simulink model "step2-part3"  (R2020b)
settings: Solver=VariableStepAuto  StartTime=0.0  StopTime=20  RelTol=1e-3
libraries: dspsnks4 x1, dspsrcs4 x1, dspvision x1, dspadpt3 x1
settings Model: Creator=berkt  LastModifiedBy=berkt

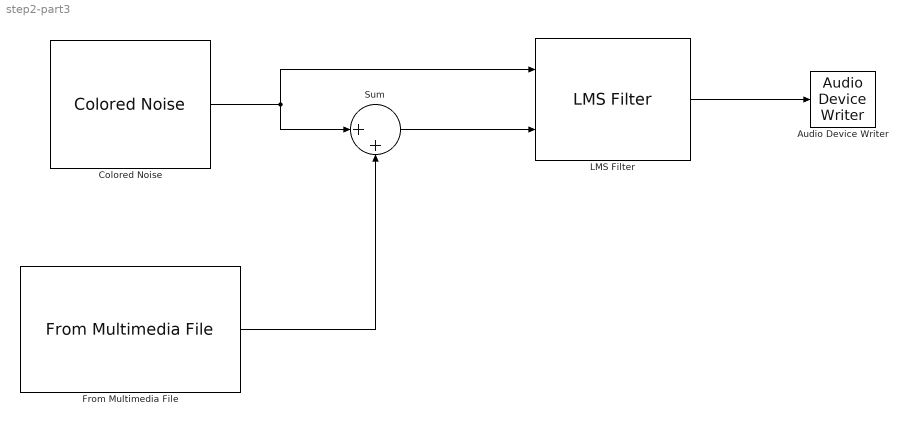
== system step2-part3 ==
  Audio Device Writer : dspsnks4/Audio Device Writer  Driver=DirectSound  Device=Default  InheritSampleRate=on  SampleRate=44100  BitDepth=16-bit integer  BufferSize=4096  NumBuffers=10  DefaultOutputChannelMapping=on  OutputChannelMapping=1:2  OutputNumUnderrunSamples=off  DriverIdx=1  DeviceWarnFlag=''
  Colored Noise : dspsrcs4/Colored Noise  Color=pink  InverseFrequencyPower=1  BoundedOutput=on  NumChannels=1  OutputDataType=double  SamplesPerFrame=1024  SampleTime=1  RandomStream=mt19937ar with seed  Seed=67  SimulateUsing=Interpreted execution
      settings: SourceProductName=DSP System Toolbox
  From Multimedia File : dspvision/From Multimedia File  inputFilename=speech_dft.mp3  readRange=[1 Inf]  loop=on  numPlays=inf  outputStreams=Audio only  videoDataType=single  audioDataType=double  inheritSampleTime=on  userDefinedSampleTime=1/30  noAudioOutput=off  isIntensityVideo=off  fourcc=RGB  colorVideoFormat=Separate color signals  outputEOF=off  dataOrg=Column-major  audioFrameSize=1024  computeAudioFrameSize=off  outSamplingMode=Sample based
  LMS Filter : dspadpt3/LMS Filter  Algo=Normalized LMS  L=32  stepflag=Dialog  mu=0.001  leakage=1.0  ic=0  Adapt=off  resetflag=None  weights=on  addnparflag=off  roundingMode=Floor  overflowMode=off
      settings: SourceProductBaseCode=DS
  Sum : Sum  Inputs=|++
  wires:
  From Multimedia File/1 -> Sum/2
  Colored Noise/1 -> LMS Filter/1, Sum/1
  Sum/1 -> LMS Filter/2
  LMS Filter/2 -> Audio Device Writer/1
